simulink library "Load_from_File"  (Simulink 8.2)
settings: Solver=ode45  StartTime=0.0  StopTime=10.0  RelTol=1e-3
undefined symbols (not defined in the file): t_sample
settings Model: Creator=lena.frank  LastModifiedBy=drhf

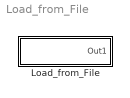
== system Load_from_File ==
  Load_from_File : Subsystem  mask(Load from File){file=FileName, ext=.mat}
      mask prompts: file "Name of file"; ext "Extension of file"
      mask help:
      | Input block for external load data files. The file is read to the workspace. A "From Workspace" Block is used in the subsystem.
      | A Unit-Delay with the timestep of the data forces the model to a maximum timestep equal to the data acquisiton timestep.
      mask init:
      | parampath = '';
      | CarnotCallbacks_GetFiles;
      | 
      | %if evalin('base',['exist (''' filename ext ''',''file'');'])
      | %    evalin('base',[filename '= importdata(''' filename ext ''');']);
      | %end
      | % set_param([gcb '/Data_from_Workspace'], 'VariableName', filename);
      | % sample time is timestep of weather data
      | % evalin('caller',['t_sample = ' filename '(3,1) - ' filename '(2,1);']);
      mask Help: web(fullfile(path_carnot('help'),'Load_from_file.html'),'-helpbrowser')
      mask TypeOptions ext: .dat | .txt | .mat
      mask Display: disp(file)

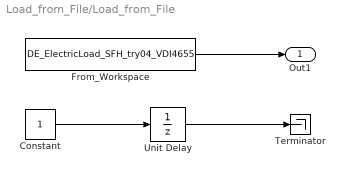
== system Load_from_File/Load_from_File ==
  Constant : Constant
  From_Workspace : FromWorkspace  VariableName=DE_ElectricLoad_SFH_try04_VDI4655  SampleTime=0
  Terminator : Terminator
  Unit Delay : UnitDelay  SampleTime=t_sample
  Out1 : Outport
  wires:
  From_Workspace/1 -> Out1/1
  Constant/1 -> Unit Delay/1
  Unit Delay/1 -> Terminator/1
